simulink model "test"  (R2021b)
settings: Solver=ode4  StartTime=0.0  StopTime=inf  FixedStep=sampleTime_control  RelTol=1e-3
undefined symbols (not defined in the file or in its folder): number, sampleTime_base, sampleTime_control
libraries: aerolibanimutils x1
settings Model: Creator=huangjlei  LastModifiedBy=huangjlei

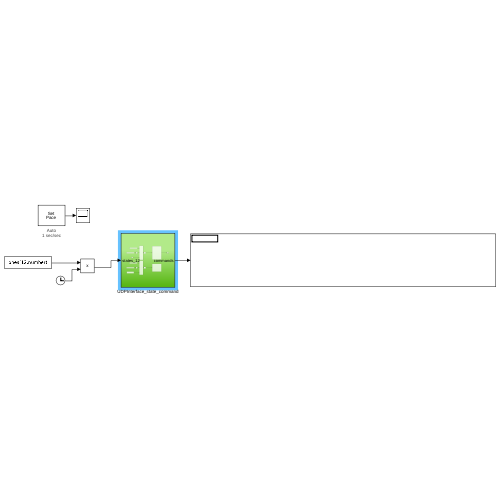
[thumbnail: Simulink's stored preview of the top-level diagram]
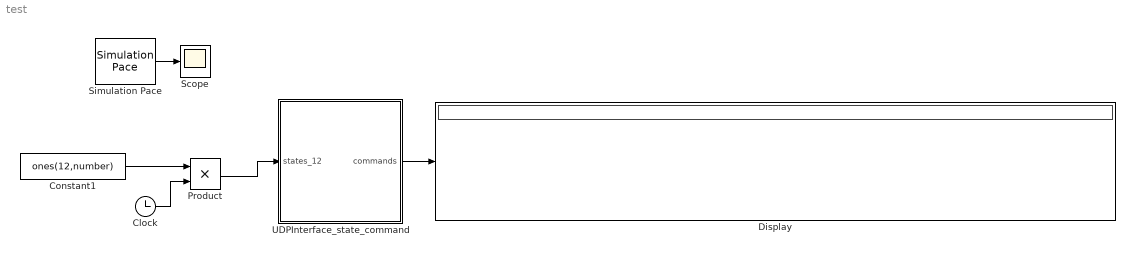
== system test ==
  Clock : Clock
  Constant1 : Constant  Value=ones(12,number)
  Display : Display
  Product : Product
  Scope : Scope
  Simulation Pace : aerolibanimutils/Simulation Pace  SimulationPace=1  SleepMode=Auto  OutputPaceError=on  SampleTime=sampleTime_base
  UDPInterface_state_command : Subsystem
  wires:
  Simulation Pace/1 -> Scope/1
  Clock/1 -> Product/2
  Constant1/1 -> Product/1
  Product/1 -> UDPInterface_state_command/1(states_12)
  UDPInterface_state_command/1(commands) -> Display/1

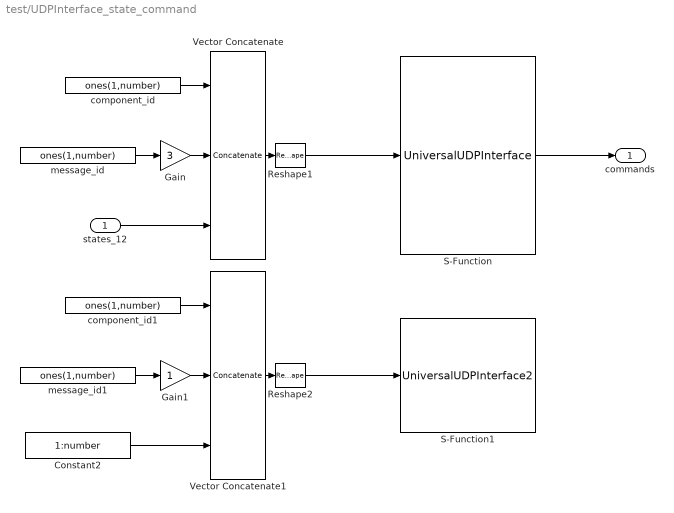
== system test/UDPInterface_state_command ==
  states_12 : Inport
  Constant2 : Constant  Value=1:number  VectorParams1D=off
  Gain : Gain  Gain=3
  Gain1 : Gain
  Reshape1 : Reshape
  Reshape2 : Reshape
  S-Function : S-Function  FunctionName=UniversalUDPInterface  Parameters=sampleTime,number,portTarget,portLocal,ipTarget,ipLocal,flagSend,flagRecv,inputPortWidth,outputPortWidth  SFunctionDeploymentMode=off  EnableBusSupport=off  mask{number=number, ipLocal=127.0.0.1, ipTarget=ones(1,number)*1, portTarget=20999, portLocal=21001, flagSend=on, flagRecv=on, inputPortWidth=14, outputPortWidth=9, sampleTime=sampleTime_control}
      mask prompts: number "Number of vehicles"; ipLocal "Local ip"; ipTarget "Target ip"; portTarget "Start port of target"; portLocal "Start port of local"; flagSend "Enable sender"; flagRecv "Enable receiver"; inputPortWidth "Width of input port"; outputPortWidth "Width of output port"; sampleTime "Sample time"
      mask help:
      | input port: componentId, messageId, msgData[0], msgData[1], ...
      | output port: systemId, numSequence, timeStamp,msgData[0], msgData[1], ...
  S-Function1 : S-Function  FunctionName=UniversalUDPInterface2  Parameters=sampleTime,number,portTarget,portLocal,ipTarget,ipLocal,flagSend,flagRecv,inputPortWidth,outputPortWidth  SFunctionDeploymentMode=off  EnableBusSupport=off  mask{number=number, ipLocal=127.0.0.1, ipTarget=ones(1,number)*1, portTarget=19999, portLocal=22001, flagSend=on, flagRecv=off, inputPortWidth=3, outputPortWidth=9, sampleTime=sampleTime_control}
      mask prompts: number "Number of vehicles"; ipLocal "Local ip"; ipTarget "Target ip"; portTarget "Start port of target"; portLocal "Start port of local"; flagSend "Enable sender"; flagRecv "Enable receiver"; inputPortWidth "Width of input port"; outputPortWidth "Width of output port"; sampleTime "Sample time"
      mask help:
      | input port: componentId, messageId, msgData[0], msgData[1], ...
      | output port: systemId, numSequence, timeStamp,msgData[0], msgData[1], ...
  Vector Concatenate : Concatenate  NumInputs=3  Mode=Multidimensional array
  Vector Concatenate1 : Concatenate  NumInputs=3  Mode=Multidimensional array
  component_id : Constant  Value=ones(1,number)  VectorParams1D=off
  component_id1 : Constant  Value=ones(1,number)  VectorParams1D=off
  message_id : Constant  Value=ones(1,number)  VectorParams1D=off
  message_id1 : Constant  Value=ones(1,number)  VectorParams1D=off
  commands : Outport
  wires:
  Vector Concatenate/1 -> Reshape1/1
  Reshape1/1 -> S-Function/1
  component_id/1 -> Vector Concatenate/1
  message_id/1 -> Gain/1
  Gain/1 -> Vector Concatenate/2
  S-Function/1 -> commands/1
  Gain1/1 -> Vector Concatenate1/2
  message_id1/1 -> Gain1/1
  Constant2/1 -> Vector Concatenate1/3
  component_id1/1 -> Vector Concatenate1/1
  Reshape2/1 -> S-Function1/1
  Vector Concatenate1/1 -> Reshape2/1
  states_12/1 -> Vector Concatenate/3
